simulink model "Garrow_with_PI"  (R2021b)
settings: Solver=VariableStepAuto  StartTime=0.0  StopTime=112  MaxStep=0.01  RelTol=1e-3
InitFcn:
  | clear all;
  | 
  | 
  | %Path in global coordinate reference frame - X and Y
  | 
  | xRef=[
  | 57.222
  | 52.707
  | 48.874
  | 44.359
  | 39.930
  | 35.160
  | 31.071
  | 16.591
  | 7.391
  | -2.575
  | -9.901
  | -13.563
  | -16.289
  | -17.567
  | -15.437
  | -8.538
  | -2.745
  | 1.002
  | 6.624
  | 10.628
  | 15.654
  | 20.935
  | 24.853
  | 28.260
  | 31.327
  | 33.797
  | 35.841
  | 36.182
  | 35.671
  | 34.478
  | 32.008
  | 29.964
  | 28.005
  | 26.301
  | 25.109
  | 24.001
  | 23.149
  | 22.383
  | 21.957
  | 21.531
  | 21.190
  | 20.850
  | 20.594
  | 21.105
  | 21.531
  | 21.701
  | 21.701
  | 21.531
  | 21.361
  | 21.446
  | 22.042
  | 23.831
  | 25.875
  | 28.771
  | ... (+154 lines)
libraries: autolibutils x4, autolibshared x2, sim3dlib x2, vehdynlibviscommon x1, slpidlib x1, simulink x1, vdynlib x1, vehdynlibsteering x1, eeGeneralControl x1, dspvision x1
(part 3 of 3)

== matlab function Garrow_with_PI/MATLAB Function ==
  data: xRef input; yRef input; yawRef input; x_actual input; y_actual input; pose input; velocity input; lookahead1_gain input; lookahead2_gain input; Steering_Angle output; Steering_ratio input
function Steering_Angle    = compute(xRef, yRef,yawRef, x_actual, y_actual, pose,velocity, lookahead1_gain, lookahead2_gain,Steering_ratio)

lookahead1=lookahead1_gain*velocity;
lookahead2=lookahead2_gain*velocity;
xcenter = 0;
ycenter = 0;

x_shifted=xRef-x_actual;
y_shifted=yRef-y_actual;

deg=360-((180/3.14)*pose);
matrix=[cosd(deg) -sind(deg);
        sind(deg) cosd(deg)];
K=cat(2,x_shifted,y_shifted);
K=K';
transformed=matrix*K;
x_path=transformed(1,:)-1.135;
y_path=transformed(2,:);
yaw_path=yawRef-pose;

distance_nearest = ((x_path.^2) +(y_path.^2)).^(0.5);
[~, index_nearest] = min(distance_nearest);
psi_error=yaw_path(index_nearest);

distance = sqrt(x_path(index_nearest:end).^2 + y_path(index_nearest:end).^2); %finds chord length to each point

difference1 = distance - lookahead1; %finds difference of chord lengths to lookahead
[~, index] = min(abs(difference1)); %finds index and value of minimum difference
x_target_1 = x_path(index+index_nearest); % finds X axis target value based on closest point to look ahead
y_target_1 = y_path(index+index_nearest); % finds y axis target value based on closest point to look ahead


difference2 = distance - lookahead2; %finds difference of chord lengths to lookahead
[~, index2] = min(abs(difference2)); %finds index and value of minimum difference
x_target_2 = x_path(index2+index_nearest); % finds X axis target value based on closest point to look ahead
y_target_2 = y_path(index2+index_nearest); % finds y axis target value based on closest point to look ahead


x1 = 0;
y1 = 0;
x2 = x_target_2;
y2 = y_target_2;
x3 = x_target_1;
y3 = y_target_1;

m12 = (y2 - y1)/(x2 - x1);
m23 = (y3 - y2)/(x3 - x2);   
xm12 = (x1+x2)/2;
ym12 = (y1+y2)/2;
xm23 = (x3+x2)/2;
ym23 = (y3+y2)/2;
mp12 = -1/m12;
mp23 = -1/m23;
% finds y intercept of each perpendicular mid line
bp12 = ym12 - mp12*xm12;
bp23 = ym23 - mp23*xm23;
% finds centerpoint coordinates
xcenter = (bp23 - bp12)/(mp12 - mp23);
ycenter = mp12*xcenter + bp12;
% finds tangent slope and calculates angle
    center_slope = ycenter/xcenter; %finds the slope of the radius from the vehicle
    target_slope = -1/center_slope; %finds the slope of the tangent line to the circle through the center of the vehicles front axle
    road_steering_angle = atan(target_slope); %calculates angle of the tangent line to the x axis to determine steering angle

Steering_Angle=(road_steering_angle+psi_error)*Steering_ratio;
end

== matlab function Garrow_with_PI/Path_smoothing_function ==
  data: u1 input; xRef output; u2 input; yRef output; yawRef output
function [xRef,yRef,yawRef] = fcn(u1,u2)

yaw=zeros(size(u1));
directionRef=ones(size(u1));
refPoses=[u1 u2 yaw];
refDirections=[directionRef];
numSmoothPoses=4500;
[poses,~] = smoothPathSpline(refPoses,refDirections,numSmoothPoses);

xRef=poses(:,1);
yRef=poses(:,2);
yawRef=poses(:,3);
yawRef=unwrap(pi*yawRef/180);

end
